simulink model "Project5"  (R2019b)
settings: Solver=ode45  StartTime=0.0  StopTime=3600  RelTol=1e-3  EnableMultiTasking=on
undefined symbols (not defined in the file): i, OCV, Q, R_Charging, SOC
settings Model: Creator=DZR3QN  LastModifiedBy=hp
settings DataIOCC: LimitDataPoints=on  SaveFormat=Array  ReturnWorkspaceOutputs=off
settings OptimizationCC: LifeSpan=inf
settings DebuggingCC: SolverPrmCheckMsg=warning  SFUnexpectedBacktrackingDiag=warning  SFNoUnconditionalDefaultTransitionDiag=warning  SFExecutionAtInitializationDiag=none  ArithmeticOperatorsInVariantConditions=warning
settings HardwareCC: ProdBitPerPointer=32  ProdBitPerSizeT=32  ProdBitPerPtrDiffT=32  ProdLargestAtomicFloat=None  ProdIntDivRoundTo=Undefined  ProdEndianess=Unspecified  ProdWordSize=32  ProdHWDeviceType=32-bit Generic
settings ModelReferenceCC: PropagateSignalLabelsOutOfModel=off
settings SFSimCC: SimUseLocalCustomCode=off  CustomCodeUndefinedFunction=UseInterfaceOnly
settings RTWCC: RTWUseLocalCustomCode=off
settings CodeAppCC: StateflowObjectComments=on
settings GRTTargetCC: TargetLangStandard=C89/C90 (ANSI)  GeneratePreprocessorConditionals=Disable all
settings ConfigComp: CovMetricSettings=dw  CovHtmlReporting=on  CovSaveCumulativeToWorkspaceVar=on  CovSaveSingleToWorkspaceVar=on  CovExternalEMLEnable=off  CovSFcnEnable=off

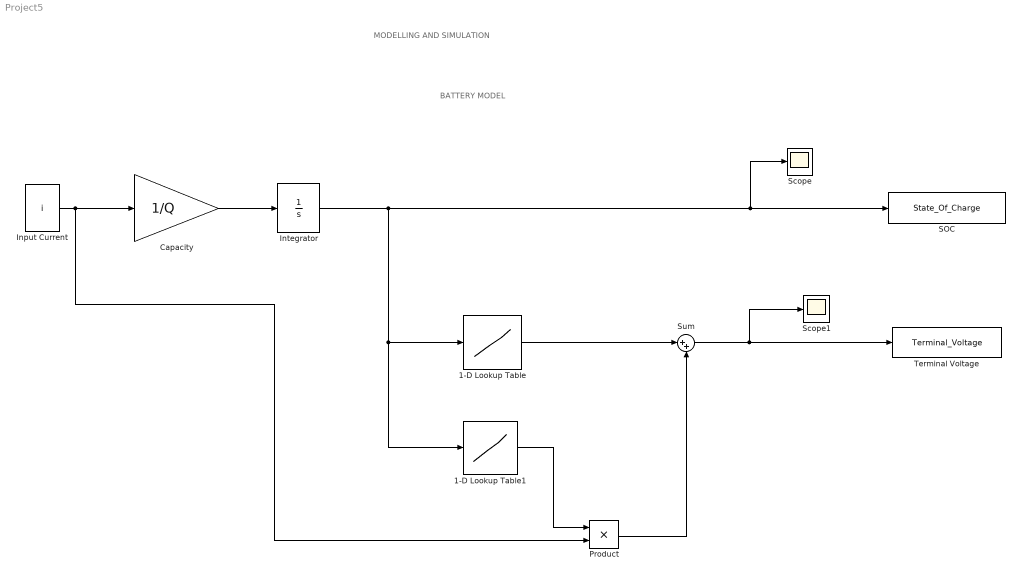
== system Project5 ==
  note: MODELLING AND SIMULATION
  note: BATTERY MODEL
  1-D Lookup Table : Lookup_n-D  NumberOfTableDimensions=1  BreakpointsForDimension1=SOC  Table=OCV  InternalRulePriority=Speed  RndMeth=Simplest  InputSameDT=on
  1-D Lookup Table1 : Lookup_n-D  NumberOfTableDimensions=1  BreakpointsForDimension1=SOC  Table=R_Charging  InternalRulePriority=Speed  RndMeth=Simplest  InputSameDT=on
  Capacity : Gain  Gain=1/Q
  Input Current : Constant  Value=i
  Integrator : Integrator
  Product : Product  RndMeth=Zero
  SOC : ToWorkspace  VariableName=State_Of_Charge  SaveFormat=Structure  SampleTime=-1
  Scope : Scope
  Scope1 : Scope
  Sum : Sum  Inputs=|++
  Terminal Voltage : ToWorkspace  VariableName=Terminal_Voltage  SaveFormat=Structure  SampleTime=-1
  wires:
  Capacity/1 -> Integrator/1
  Input Current/1 -> Product/2, Capacity/1
  Integrator/1 -> 1-D Lookup Table1/1, 1-D Lookup Table/1, Scope/1, SOC/1
  1-D Lookup Table1/1 -> Product/1
  Product/1 -> Sum/2
  1-D Lookup Table/1 -> Sum/1
  Sum/1 -> Scope1/1, Terminal Voltage/1
